simulink model "slb_ROM_LUT_Sin"  (R2015b)
settings: Solver=ode45  SolverMode=SingleTasking  StartTime=0.0  StopTime=520/2000  RelTol=1e-3
undefined symbols (not defined in the file): j
libraries: simulink x2, dspsigops x1
settings Model: Creator=amatsumo  LastModifiedBy=amatsumo
settings DataIOCC: SaveFormat=Array  SignalLoggingSaveFormat=ModelDataLogs  SaveOutput=off  SignalLogging=off  SaveTime=off
settings OptimizationCC: BlockReduction=off  ConditionallyExecuteInputs=off  DefaultParameterBehavior=Inlined  ExpressionDepthLimit=2147483647
settings DebuggingCC: AlgebraicLoopMsg=error  UnderspecifiedInitializationDetection=Classic  MergeDetectMultiDrivingBlocksExec=none  SolverPrmCheckMsg=warning  InheritedTsInSrcMsg=none  SingleTaskRateTransMsg=error  FcnCallInpInsideContextMsg=UseLocalSettings  StateNameClashWarn=warning
settings HardwareCC: ProdBitPerPointer=32  ProdLargestAtomicFloat=None  ProdIntDivRoundTo=Undefined  ProdEndianess=Unspecified  ProdWordSize=32  ProdHWDeviceType=ASIC/FPGA->ASIC/FPGA  ProdEqTarget=off
settings SFSimCC: SimParseCustomCode=off
settings GRTTargetCC: GeneratePreprocessorConditionals=Disable all  CombineOutputUpdateFcns=off  GRTInterface=on
settings ConfigComp: CovModelRefEnable=Off  CovSFcnEnable=off

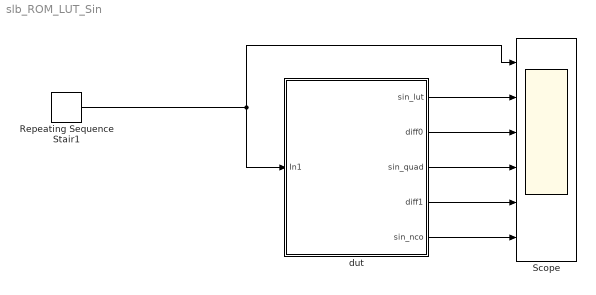
== system slb_ROM_LUT_Sin ==
  Repeating Sequence Stair1 : simulink/Sources/Repeating Sequence Stair  OutValues=0:255  tsamp=1/2000  OutMin=[]  OutMax=[]  OutDataTypeStr=fixdt(0,8,0)  OutputDataTypeScalingMode=Specify via dialog  OutDataType=fixdt(0,8,0)  ConRadixGroup=Best Precision: Vector-wise  OutScaling=[]
  Scope : Scope  NumInputPorts=6
  dut : Subsystem
  wires:
  Repeating Sequence Stair1/1 -> Scope/1, dut/1(In1)
  dut/4(diff1) -> Scope/5
  dut/3(sin_quad) -> Scope/4
  dut/5(sin_nco) -> Scope/6
  dut/2(diff0) -> Scope/3
  dut/1(sin_lut) -> Scope/2

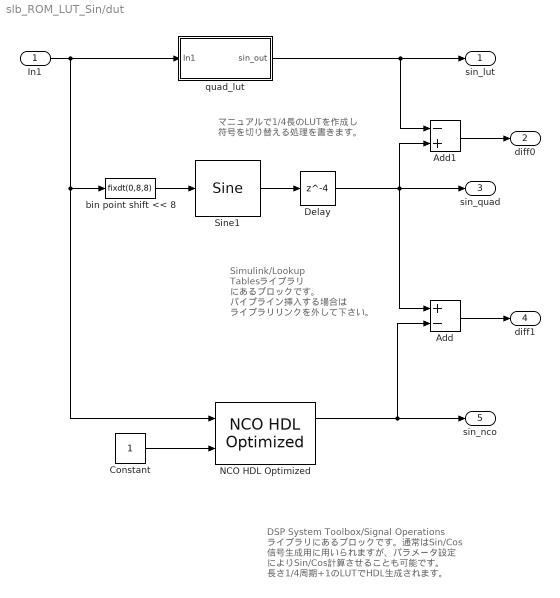
== system slb_ROM_LUT_Sin/dut ==
  note: DSP System Toolbox/Signal Operations
      | ライブラリにあるブロックです。通常はSin/Cos
      | 信号生成用に用いられますが、パラメータ設定
      | によりSin/Cos計算させることも可能です。
      | 長さ1/4周期+1のLUTでHDL生成されます。
  note: Simulink/Lookup Tablesライブラリ
      | にあるブロックです。
      | パイプライン挿入する場合は
      | ライブラリリンクを外して下さい。
  note: マニュアルで1/4長のLUTを作成し
      | 符号を切り替える処理を書きます。
  In1 : Inport
  Add : Sum  Inputs=+-
  Add1 : Sum  Inputs=-+
  Constant : Constant  OutDataTypeStr=boolean  SampleTime=-1
  Delay : Delay  DelayLength=4
  NCO HDL Optimized : dspsigops/NCO HDL Optimized  PhaseIncrementSource=Property  PhaseIncrement=0  PhaseOffsetSource=Input port  PhaseOffset=0  DitherSource=Property  NumDitherBits=2  PhaseQuantization=on  NumQuantizerAccumulatorBits=8  LUTCompress=on  ResetAction=off  ValidInputPort=on  Waveform=Sine  PhasePort=off  AccumulatorWL=16  OutputDataType=Binary point scaling  OutputWL=16  OutputFL=14  SimulateUsing=Code generation
  Sine1 : simulink/Lookup Tables/Sine  Formula=sin(2*pi*u)  NumDataPoints=(2^6)+1  OutputWordLength=16  InternalRulePriority=Speed
  bin point shift << 8 : DataTypeConversion  OutDataTypeStr=fixdt(0,8,8)  ConvertRealWorld=Stored Integer (SI)  RndMeth=Nearest
  quad_lut : Subsystem
  sin_lut : Outport
  diff0 : Outport  Port=2
  sin_quad : Outport  Port=3
  diff1 : Outport  Port=4
  sin_nco : Outport  Port=5
  wires:
  quad_lut/1(sin_out) -> Add1/1, sin_lut/1
  In1/1 -> NCO HDL Optimized/1, bin point shift << 8/1, quad_lut/1(In1)
  Delay/1 -> Add/1, Add1/2, sin_quad/1
  NCO HDL Optimized/1 -> sin_nco/1, Add/2
  Sine1/1 -> Delay/1
  Add1/1 -> diff0/1
  Add/1 -> diff1/1
  Constant/1 -> NCO HDL Optimized/2
  bin point shift << 8/1 -> Sine1/1

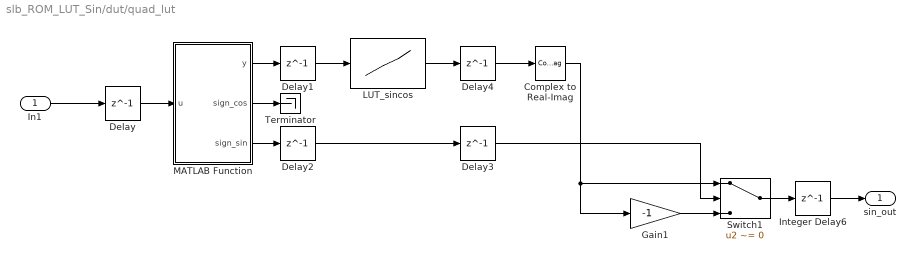
== system slb_ROM_LUT_Sin/dut/quad_lut ==
  In1 : Inport
  Complex to Real-Imag : ComplexToRealImag  Output=Imag
  Delay{,1..4} (5 alike) : Delay  DelayLength=1
  Gain1 : Gain  Gain=-1  ParamDataTypeStr=fixdt(1,2,0)  OutDataTypeStr=Inherit: Same as input
  Integer Delay6 : Delay  DelayLength=1
  LUT_sincos : Lookup_n-D  NumberOfTableDimensions=1  BreakpointsForDimension1=0:64  IndexSearchMethod=Evenly spaced points  Table=exp(j*2*pi*(0:64)/256)  InterpMethod=Flat  ExtrapMethod=Clip  UseLastTableValue=on  OutDataTypeStr=fixdt(1,16,14)  RndMeth=Simplest  InputSameDT=on  LockScale=on
  MATLAB Function : MATLAB Function  TreatAsAtomicUnit=on
  Switch1 : Switch  Criteria=u2 ~= 0
  Terminator : Terminator
  sin_out : Outport
  wires:
  LUT_sincos/1 -> Delay4/1
  In1/1 -> Delay/1
  Delay/1 -> MATLAB Function/1(u)
  MATLAB Function/1(y) -> Delay1/1
  Delay1/1 -> LUT_sincos/1
  MATLAB Function/2(sign_cos) -> Terminator/1
  Delay4/1 -> Complex to Real-Imag/1
  Complex to Real-Imag/1 -> Gain1/1, Switch1/1
  Switch1/1 -> Integer Delay6/1
  Integer Delay6/1 -> sin_out/1
  Gain1/1 -> Switch1/3
  MATLAB Function/3(sign_sin) -> Delay2/1
  Delay2/1 -> Delay3/1
  Delay3/1 -> Switch1/2

== matlab function slb_ROM_LUT_Sin/dut/quad_lut/MATLAB Function ==
  data: u input; y output; sign_cos output boolean; sign_sin output
function [y, sign_cos, sign_sin] = fcn(u)
%#codegen
numType = numerictype(0,7,0);

if (u>=0 && u < 64)
	sign_cos = true;
	sign_sin = true;
	y = fi(u,numType);
elseif (u >= 64 && u < 128)
	sign_cos = false;
	sign_sin = true;
	y = fi(128-u,numType);
elseif (u >= 128 && u < 192)
	sign_cos = false;
	sign_sin = false;
	y = fi(u-128,numType);
else	% u >= 192 && u < 255
	sign_cos = true;
	sign_sin = false;
	tmp = fi(fi(256, 1, 10, 0)-u,1, 9, 0);	
	y = fi(tmp,numType);	
end
